simulink model "model_suspentionsystem"  (R2016a)
settings: Solver=ode1  StartTime=0.0  StopTime=7  FixedStep=0.01  RelTol=1e-3
settings Model: Creator=ALA  LastModifiedBy=ALA

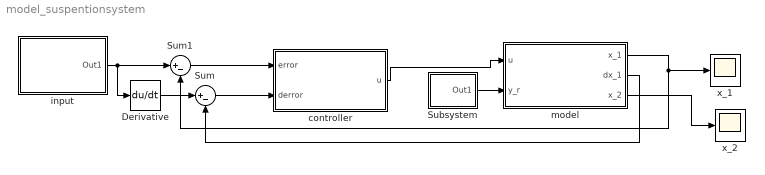
== system model_suspentionsystem ==
  Derivative : Derivative
  Subsystem : Subsystem
  Sum : Sum  Inputs=|+-
  Sum1 : Sum  Inputs=|+-
  controller : Subsystem
  "input " : Subsystem
  model : Subsystem
  x_1 : Scope
  x_2 : Scope
  wires:
  controller/1(u) -> model/1(u)
  model/1(x_1) -> Sum1/2, x_1/1
  "input "/1(Out1) -> Derivative/1, Sum1/1
  Sum1/1 -> controller/1(error)
  Derivative/1 -> Sum/1
  Sum/1 -> controller/2(derror)
  model/2(dx_1) -> Sum/2
  Subsystem/1(Out1) -> model/2(y_r)
  model/3(x_2) -> x_2/1

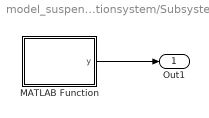
== system model_suspentionsystem/Subsystem ==
  MATLAB Function : MATLAB Function  TreatAsAtomicUnit=on
  Out1 : Outport
  wires:
  MATLAB Function/1(y) -> Out1/1

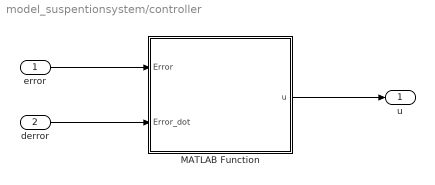
== system model_suspentionsystem/controller ==
  error : Inport
  derror : Inport  Port=2
  MATLAB Function : MATLAB Function  TreatAsAtomicUnit=on
  u : Outport
  wires:
  error/1 -> MATLAB Function/1(Error)
  MATLAB Function/1(u) -> u/1
  derror/1 -> MATLAB Function/2(Error_dot)

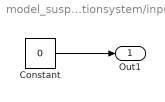
== system model_suspentionsystem/input  ==
  Constant : Constant  Value=0
  Out1 : Outport
  wires:
  Constant/1 -> Out1/1

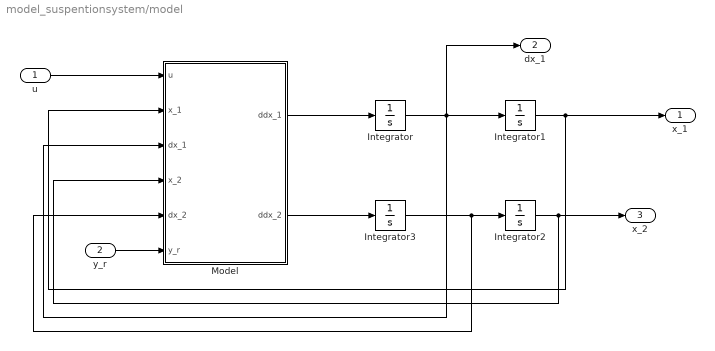
== system model_suspentionsystem/model ==
  u : Inport
  y_r : Inport  Port=2
  Integrator : Integrator
  Integrator1 : Integrator  InitialCondition=0.2
  Integrator2 : Integrator
  Integrator3 : Integrator
  Model : MATLAB Function  TreatAsAtomicUnit=on
  x_1 : Outport
  dx_1 : Outport  Port=2
  x_2 : Outport  Port=3
  wires:
  u/1 -> Model/1(u)
  Integrator/1 -> dx_1/1, Model/3(dx_1), Integrator1/1
  Model/1(ddx_1) -> Integrator/1
  Model/2(ddx_2) -> Integrator3/1
  Integrator3/1 -> Model/5(dx_2), Integrator2/1
  Integrator1/1 -> Model/2(x_1), x_1/1
  Integrator2/1 -> x_2/1, Model/4(x_2)
  y_r/1 -> Model/6(y_r)

== matlab function model_suspentionsystem/controller/MATLAB Function ==
  data: Error input; u output; Error_dot input
%------------controller------------------
%           suspention system cotroll
%          (c)copyright 2020,Isfahan University of Technology
%           all rights reserved
% file:
% By:Ala Bazazzadeh   student No.:9638403
% version:
% description:This is a PD-controller designed to decrease the turbulance
% in vihicle's cabin.
%----------------------------------------

function u=fcn(Error,Error_dot)
%-------------vriable configuration-------
kp=550;   %proportional factor
kd=550;   % drived factor 
%-------------PD controller equation------ 
u = kp*Error + kd*Error_dot;

== matlab function model_suspentionsystem/model/Model ==
  data: u input; x_1 input; dx_1 input; x_2 input; dx_2 input; y_r input; ddx_1 output; ddx_2 output
%------------model------------------
%           suspention system cotroll
%          (c)copyright 2020,Isfahan University of Technology
%           all rights reserved
% file:
% By:Ala Bazazzadeh   student No.:9638403
% version:1.1.1
% description:this is the main part of the suspention system named model
%-----------------------------------
function [ddx_1,ddx_2] = fcn(u,x_1,dx_1,x_2,dx_2,y_r)

%-----------parameters---------------
M=300;   %mass of vihicle Kg
m=50;    %mass of suspention system Kg
k_1=300;  %spring No.1's costant N/m
k_2=30000; %spring No.2's costant N/m
D=600;     %damper's costant

%-----------dynamic equations--------

ddx_1 =(1/M)*(u-(k_1)*(x_1-x_2)-D*(dx_1-dx_2));
ddx_2 =(1/m)*(-u-(k_1)*(x_2-x_1)-D*(dx_2-dx_1)-(k_2)*(x_2 - y_r));

== matlab function model_suspentionsystem/Subsystem/MATLAB Function ==
  data: y output
function y = fcn()
 for i=0:4
     for(t=0:7)
     y=0.1*(sin(5+4*i)*t);
     end
 end
